simulink model "simulink_ld"  (R2018a)
settings: Solver=VariableStepAuto  StartTime=0.0  StopTime=500  RelTol=1e-3
values from neighbouring files (symbols this model uses):
  ae = 329.2  / fator    (= 5.48666666667)    [carregaDadosDoModelo.m]    (also in carregaDadosSimulacao.m = 5.4867)
  anp = 16.5    [carregaDadosSimulacao.m]
  av = 414.17 / fator    (= 6.90283333333)    [carregaDadosDoModelo.m]    (also in carregaDadosSimulacao.m = 6.9028)
  K = 0.36783    [carregaDados.m]    (also in carregaDadosDoModelo.m = 0.01332; carregaDadosSimulacao.m = 0.01)
  Kc = 1       * fator    (= 60)    [carregaDadosDoModelo.m]    (also in carregaDadosSimulacao.m = 2.5)
  Ke = 0.395   * fator    (= 23.7)    [carregaDadosDoModelo.m]    (also in carregaDadosSimulacao.m = 1.4)
  Knp = 0.1    [carregaDadosSimulacao.m]
  Kr = 0.016835* fator    (= 1.0101)    [carregaDadosDoModelo.m]
  Ktp = 36.5    [carregaDadosSimulacao.m]
  Kv = 0.647   * fator    (= 38.82)    [carregaDadosDoModelo.m]    (also in carregaDadosSimulacao.m = 3.3)
  td = 0.065    [carregaDados.m]    (also in carregaDadosSimulacao.m = 5)
settings Model: Creator=alexa  LastModifiedBy=alexa

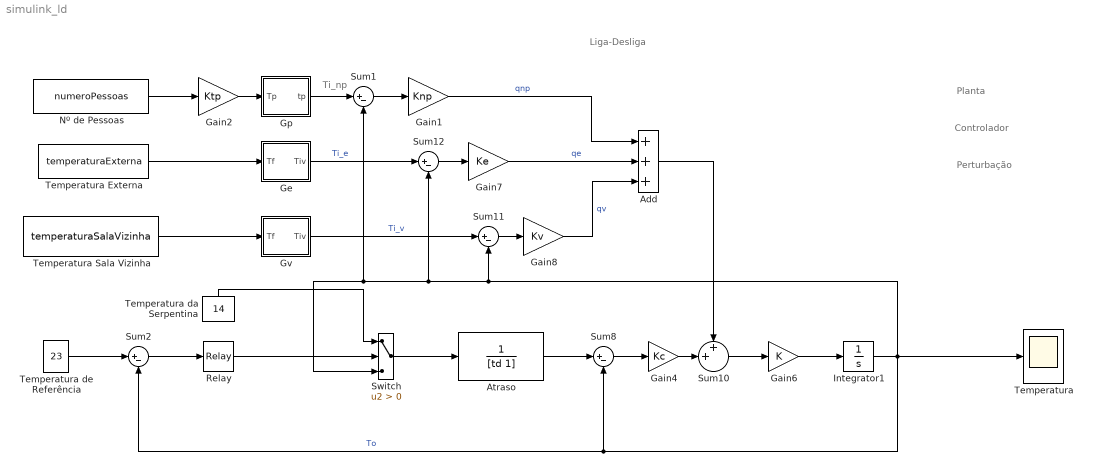
== system simulink_ld ==
  note: Liga-Desliga
  note: Perturbação
  note: Planta
  note: Ti_np
  note: Controlador
  Add : Sum  Inputs=+++
  Atraso : TransferFcn  Denominator=[td 1]
  Gain1 : Gain  Gain=Knp
  Gain2 : Gain  Gain=Ktp
  Gain4 : Gain  Gain=Kc
  Gain6 : Gain  Gain=K
  Gain7 : Gain  Gain=Ke
  Gain8 : Gain  Gain=Kv
  Ge : Subsystem
  Gp : Subsystem
  Gv : Subsystem
  Integrator1 : Integrator  InitialCondition=30
  Nº de Pessoas : FromWorkspace  VariableName=numeroPessoas  SampleTime=1
  Relay : Relay  OnSwitchValue=0.3  OffSwitchValue=-0.3  OnOutputValue=0  OffOutputValue=1
  Sum{1..2,8,11..12} (5 alike) : Sum  Inputs=|+-
  Sum10 : Sum  Inputs=++|
  Switch : Switch  Criteria=u2 > Threshold
  Temperatura : Scope
  Temperatura da Serpentina : Constant  Value=14
  Temperatura de Referência : Constant  Value=23
  Temperatura Externa : FromWorkspace  VariableName=temperaturaExterna  SampleTime=1
  Temperatura Sala Vizinha : FromWorkspace  VariableName=temperaturaSalaVizinha  SampleTime=1
  wires:
  Atraso/1 -> Sum8/1
  Sum12/1 -> Gain7/1
  Gp/1("tp ") -> Sum1/1
  Gain6/1 -> Integrator1/1
  Nº de Pessoas/1 -> Gain2/1
  Gain2/1 -> Gp/1(Tp)
  Switch/1 -> Atraso/1
  Gain8/1 -> Add/3  "qv"
  Gv/1(Tiv) -> Sum11/1  "Ti_v"
  Temperatura da Serpentina/1 -> Switch/1
  Add/1 -> Sum10/1
  Sum8/1 -> Gain4/1
  Ge/1(Tiv) -> Sum12/1  "Ti_e"
  Temperatura Sala Vizinha/1 -> Gv/1(Tf)
  Sum10/1 -> Gain6/1
  Sum11/1 -> Gain8/1
  Sum1/1 -> Gain1/1
  Gain7/1 -> Add/2  "qe"
  Relay/1 -> Switch/2
  Temperatura Externa/1 -> Ge/1(Tf)
  Gain1/1 -> Add/1  "qnp"
  Gain4/1 -> Sum10/2
  Integrator1/1 -> Sum2/2, Sum8/2, Temperatura/1, Switch/3, Sum1/2, Sum12/2, Sum11/2  "To"
  Temperatura de Referência/1 -> Sum2/1
  Sum2/1 -> Relay/1

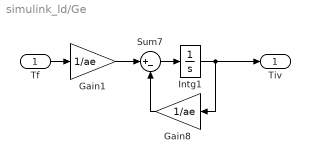
== system simulink_ld/Ge ==
  Tf : Inport
  Gain1 : Gain  Gain=1/ae
  Gain8 : Gain  Gain=1/ae
  Intg1 : Integrator  InitialCondition=30
  Sum7 : Sum  Inputs=|+-
  Tiv : Outport
  wires:
  Gain1/1 -> Sum7/1
  Tf/1 -> Gain1/1
  Gain8/1 -> Sum7/2
  Intg1/1 -> Tiv/1, Gain8/1
  Sum7/1 -> Intg1/1

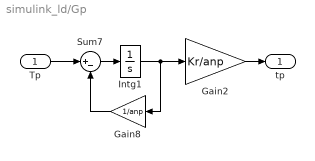
== system simulink_ld/Gp ==
  Tp : Inport
  Gain2 : Gain  Gain=Kr/anp
  Gain8 : Gain  Gain=1/anp
  Intg1 : Integrator
  Sum7 : Sum  Inputs=|+-
  "tp " : Outport
  wires:
  Gain2/1 -> "tp "/1
  Tp/1 -> Sum7/1
  Gain8/1 -> Sum7/2
  Intg1/1 -> Gain2/1, Gain8/1
  Sum7/1 -> Intg1/1

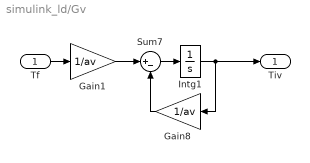
== system simulink_ld/Gv ==
  Tf : Inport
  Gain1 : Gain  Gain=1/av
  Gain8 : Gain  Gain=1/av
  Intg1 : Integrator  InitialCondition=30
  Sum7 : Sum  Inputs=|+-
  Tiv : Outport
  wires:
  Gain1/1 -> Sum7/1
  Tf/1 -> Gain1/1
  Gain8/1 -> Sum7/2
  Intg1/1 -> Tiv/1, Gain8/1
  Sum7/1 -> Intg1/1
